simulink model "PCS"  (Simulink 8.0)
settings: Solver=ode23  StartTime=0.0  StopTime=0.3  RelTol=1e-3
undefined symbols (not defined in the file or in its folder): DiscIntNeverNeededParam, Ion, Lithium
libraries: powerlib x54, simulink x4, electricdrivelib x1, powerlib_extras x1
settings Model: Creator=wzhenh  LastModifiedBy=Administrator
settings SolverCC: ZeroCrossControl=DisableAll
settings DebuggingCC: FrameProcessingCompatibilityMsg=error
settings CodeAppCC: CustomSymbolStrType=$N$R$M_T  InternalIdentifier=Shortened
settings GRTTargetCC: CodeReplacementLibrary=None  CPPClassGenCompliant=on

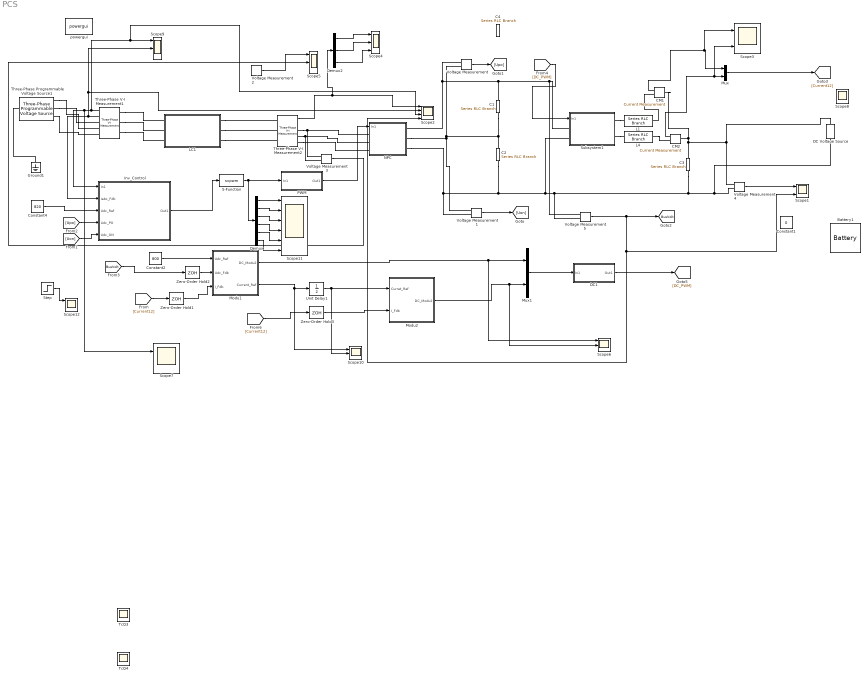
== system PCS ==
  Battery1 : electricdrivelib/Extra Sources/Battery  BatType=Lithium-Ion  ShowDetailedParameters=off  NomV=450  NomQ=2.5  SOC=20  PresetModel=off  MaxQ=2.625  FullV=2357.0739  Dis_rate=0.027175  R=1.8  Normal_OP=0.0565225  expZone=[2187.7812 0.0030706525]  Dis_Char=off  current=[1.5 3]  Units=Ampere-hour  Batt_Tr=30
  C1 : powerlib/Elements/Series RLC Branch  LConnTagsString=__new0  RConnTagsString=__new0  BranchType=C  Resistance=0.05  Inductance=22e-3  SetiL0=off  InitialCurrent=0  Capacitance=4110e-6  Setx0=on  InitialVoltage=480/1.732*1.414/2  Measurements=None
  C2 : powerlib/Elements/Series RLC Branch  LConnTagsString=__new0  RConnTagsString=__new0  BranchType=C  Resistance=0.05  Inductance=22e-3  SetiL0=off  InitialCurrent=0  Capacitance=4110e-6  Setx0=on  InitialVoltage=480/1.732*1.414/2  Measurements=None
  C3 : powerlib/Elements/Series RLC Branch  LConnTagsString=__new0  RConnTagsString=__new0  BranchType=RC  Resistance=0.05  Inductance=22e-3  SetiL0=off  InitialCurrent=0  Capacitance=120e-6  Setx0=off  InitialVoltage=400  Measurements=None
  C4 : powerlib/Elements/Series RLC Branch  LConnTagsString=__new0  RConnTagsString=__new0  BranchType=C  Resistance=0.05  Inductance=22e-3  SetiL0=off  InitialCurrent=0  Capacitance=4110e-6  Setx0=off  InitialVoltage=400  Measurements=None
  CM1 : powerlib/Measurements/Current Measurement  PhasorSimulation=off  OutputType=Complex  PSBequivalent=0
  CM2 : powerlib/Measurements/Current Measurement  PhasorSimulation=off  OutputType=Complex  PSBequivalent=0
  Constant1 : Constant  Value=0
  Constant2 : Constant  Value=800
  Constant4 : Constant  Value=820
  DC Voltage Source : powerlib/Electrical Sources/DC Voltage Source  Amplitude=450  Measurements=None
  DC1 : Subsystem
      mask init:
      | Dc_Pwm=7.8125e-6/5
  Demux : Demux  Outputs=6
  Demux2 : Demux  Outputs=3
  Ground1 : powerlib/Elements/Ground  LConnTagsString=a
  Inv_Control : Subsystem
  L1 : powerlib/Elements/Series RLC Branch  LConnTagsString=__new0  RConnTagsString=__new0  BranchType=L  Resistance=1  Inductance=1e-3  SetiL0=off  InitialCurrent=20  Capacitance=1e-6  Setx0=off  InitialVoltage=0  Measurements=None
  L4 : powerlib/Elements/Series RLC Branch  LConnTagsString=__new0  RConnTagsString=__new0  BranchType=L  Resistance=1  Inductance=1e-3  SetiL0=off  InitialCurrent=20  Capacitance=1e-6  Setx0=off  InitialVoltage=0  Measurements=None
  LC1 : Subsystem
  Modu1 : Subsystem
      mask init:
      | Ts_Dc=62.5e-6
  Modu2 : Subsystem
      mask init:
      | Ts_Dc=62.5e-6
  Mux : Mux  Inputs=2
  Mux1 : Mux  Inputs=2
  NPC : Subsystem
  PWM : Subsystem
      mask init:
      | Ts_Pwm=1.5625e-6
  S-Function : S-Function  FunctionName=svpwm  EnableBusSupport=off
  Scope{1,4..6,8..10,12} (8 alike) : Scope  NumInputPorts=3
      Scope4 settings: YMin=-5~-5~-5  YMax=5~5~5
  Scope11 : Scope  NumInputPorts=6
  Scope2 : Scope  NumInputPorts=4
      settings: YMin=-1000~-15~-400~799  YMax=1000~15~400~803.5
  Scope3 : Scope  NumInputPorts=2
      settings: YMin=-5~-5  YMax=5~5
  Scope7 : Scope  NumInputPorts=2
  Step : Step  Time=0.2  Before=780  After=820  SampleTime=62.5e-6
  Subsystem1 : Subsystem
  TcQ3 : Scope
  TcQ4 : Scope
  Three-Phase Programmable Voltage Source1 : powerlib/Electrical Sources/Three-Phase Programmable Voltage Source  PositiveSequence=[480 0 50]  VariationEntity=None  VariationType=Table of time-amplitude pairs  VariationTypeAlt=Step  VariationStep=0.5  VariationRate=10  VariationMagnitude=0.3  VariationFrequency=2  VariationTiming=[1 2]  VariationPhaseA=off  Amplitudes=[1 0.8 1.2 1.0]  TimeValues=[0 0.1 0.15 0.2]  HarmonicGeneration=off  HarmonicA=[3 0.2 -25 0]  HarmonicB=[2 0.15 35 2]  Timing="[0.05  3]"  BusType=swing  Pref=0  Qref=0  Qmin=-inf  Qmax=inf
  Three-Phase V-I Measurement1 : powerlib/Measurements/Three-Phase V-I Measurement  VoltageMeasurement=phase-to-ground  SetLabelV=off  LabelV=Vabc  Vpu=off  VpuLL=off  CurrentMeasurement=yes  SetLabelI=off  LabelI=Iabc  Ipu=off  Pbase=30000  Vbase=480  OutputType=Complex  PhasorSimulation=off  PSBequivalent=0
  Three-Phase V-I Measurement2 : powerlib/Measurements/Three-Phase V-I Measurement  VoltageMeasurement=phase-to-phase  SetLabelV=off  LabelV=Vabc  Vpu=off  VpuLL=off  CurrentMeasurement=yes  SetLabelI=off  LabelI=Iabc  Ipu=off  Pbase=30000  Vbase=480  OutputType=Complex  PhasorSimulation=off  PSBequivalent=0
  Unit Delay1 : UnitDelay  SampleTime=31.125e-6
  Voltage Measurement{,1..5} (6 alike) : powerlib/Measurements/Voltage Measurement  PhasorSimulation=off  OutputType=Complex  PSBequivalent=0
  Zero-Order Hold1 : ZeroOrderHold  SampleTime=62.5e-6
  Zero-Order Hold2 : ZeroOrderHold  SampleTime=125e-6
  Zero-Order Hold3 : ZeroOrderHold  SampleTime=62.5e-6
  powergui : powerlib/powergui  Priority=1  SimulationMode=Discrete  SolverType=Tustin  SampleTime=62.5e-6/32  frequency=60  SPID=off  DisableSnubberDevices=off  DisableRonSwitches=off  DisableVfSwitches=off  SwTol=0  Interpol=off  DisplayEquations=off  FunctionMessages=off  frequencyindice=0  Pbase=30000e3  ErrMax=1e-4  Iterations=50  UnitsV=kV  UnitsW=MW  echomessages=off  HookPort=off  EnableUseOfTLC=off  x0status=blocks  RestoreLinks=warning  ResistiveCurrentMeasurement=off  Frange=[0:2:500]  Ylog=off  Xlog=on  ShowGrid=off  save=off  variable=ZData  structure=psbbridges_str  ZoomFFT=off  StartTime=0.0  cycles=1  DisplayStyle=1  fundamental=50  FreqAxis=off  MaxFrequency=1000  frequencyindicesteady=1  RmsSteady=1  display=off  Ts=0  methode=off
  tag scope: BusVolt=global
  wires:
  Voltage Measurement/1 -> [Upo]
  Voltage Measurement1/1 -> [Uon]
  ? -> TcQ4/1
  ? -> TcQ3/1
  PWM/1(Out1) -> NPC/1(In1)
  [Uon] -> Inv_Control/5(Udc_ON)
  [Upo] -> Inv_Control/4(Udc_PO)
  Three-Phase V-I Measurement2/1 -> Demux2/1, Scope2/1
  S-Function/1 -> Demux/1, PWM/1(In1)
  Demux2/1 -> Scope4/1
  Demux2/2 -> Scope4/2
  Demux2/3 -> Scope4/3
  Voltage Measurement2/1 -> Scope5/1
  Voltage Measurement3/1 -> Scope5/2
  Inv_Control/1(Out1) -> S-Function/1
  Three-Phase V-I Measurement1/1 -> Scope2/3, Scope9/1, Scope7/1, Inv_Control/1(In1)
  Three-Phase V-I Measurement1/2 -> Scope2/2, Scope9/2, Inv_Control/2(Iabc_Fdb)
  [Current12] -> Zero-Order Hold1/1
  [Current12] -> Zero-Order Hold3/1
  Constant2/1 -> Modu1/1(Udc_Ref)
  Zero-Order Hold2/1 -> Modu1/2(Udc_Fdb)
  Zero-Order Hold1/1 -> Modu1/3(I_Fdb)
  Zero-Order Hold3/1 -> Modu2/2(I_Fdb)
  Modu1/2(Current_Ref) -> Scope10/1, Unit Delay1/1
  Unit Delay1/1 -> Modu2/1(Curret_Ref), Scope10/2
  [DC_PWM] -> Subsystem1/1(In1)
  Voltage Measurement4/1 -> Scope1/1
  Modu1/1(DC_Modu2) -> Scope6/1, Mux1/1
  Modu2/1(DC_Modu2) -> Scope6/2, Mux1/2
  Mux1/1 -> DC1/1(In1)
  DC1/1(Out1) -> [DC_PWM]
  [BusVolt] -> Zero-Order Hold2/1
  Voltage Measurement5/1 -> Scope2/4, Scope1/3, [BusVolt]
  CM1/1 -> Scope3/1, Mux/1
  CM2/1 -> Scope3/2, Mux/2
  Mux/1 -> [Current12]
  Demux/1 -> Scope11/1
  Demux/2 -> Scope11/2
  Demux/3 -> Scope11/3
  Demux/4 -> Scope11/4
  Demux/5 -> Scope11/5
  Demux/6 -> Scope11/6
  Step/1 -> Scope12/1
  Constant4/1 -> Inv_Control/3(Udc_Ref)
  connections:
  Three-Phase V-I Measurement2/RConn1 -- Voltage Measurement3/LConn1 -- NPC/LConn1
  Three-Phase V-I Measurement2/RConn2 -- Voltage Measurement3/LConn2 -- NPC/LConn2
  Ground1/LConn1 -- Three-Phase Programmable Voltage Source1/LConn1
  Three-Phase V-I Measurement2/RConn3 -- NPC/LConn3
  LC1/RConn1 -- Three-Phase V-I Measurement2/LConn1
  LC1/RConn2 -- Three-Phase V-I Measurement2/LConn2
  LC1/RConn3 -- Three-Phase V-I Measurement2/LConn3
  Three-Phase Programmable Voltage Source1/RConn1 -- Three-Phase V-I Measurement1/RConn1
  Three-Phase Programmable Voltage Source1/RConn2 -- Three-Phase V-I Measurement1/RConn2
  Three-Phase Programmable Voltage Source1/RConn3 -- Three-Phase V-I Measurement1/RConn3
  Three-Phase V-I Measurement1/LConn1 -- LC1/LConn1
  Three-Phase V-I Measurement1/LConn2 -- LC1/LConn2
  Three-Phase V-I Measurement1/LConn3 -- LC1/LConn3
  Subsystem1/RConn2 -- L4/LConn1
  Subsystem1/RConn1 -- L1/LConn1
  C3/LConn1 -- CM1/LConn1 -- CM2/LConn1 -- DC Voltage Source/RConn1 -- Voltage Measurement4/LConn1
  L1/RConn1 -- CM1/RConn1
  C1/LConn1 -- Voltage Measurement5/LConn1 -- Subsystem1/LConn1 -- NPC/RConn1 -- Voltage Measurement/LConn1
  Voltage Measurement/LConn2 -- Voltage Measurement1/LConn1 -- NPC/RConn2 -- C2/LConn1 -- C1/RConn1
  C3/RConn1 -- Subsystem1/LConn2 -- C2/RConn1 -- Voltage Measurement1/LConn2 -- NPC/RConn3 -- Voltage Measurement5/LConn2 -- DC Voltage Source/LConn1 -- Voltage Measurement4/LConn2
  L4/RConn1 -- CM2/RConn1

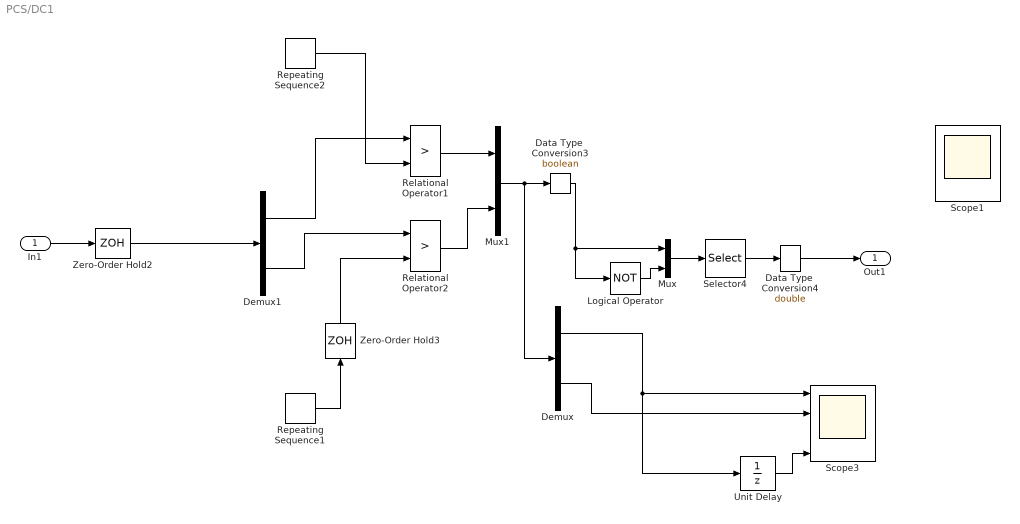
== system PCS/DC1 ==
  In1 : Inport
  Data Type  Conversion3 : DataTypeConversion  OutDataTypeStr=boolean  SampleTime=Dc_Pwm  SaturateOnIntegerOverflow=on  RndMeth=Zero
  Data Type  Conversion4 : DataTypeConversion  OutDataTypeStr=double  SampleTime=Dc_Pwm  SaturateOnIntegerOverflow=on  RndMeth=Zero
  Demux : Demux  Outputs=2
  Demux1 : Demux  Outputs=2
  Logical Operator : Logic  Operator=NOT  AllPortsSameDT=off  OutDataTypeStr=boolean  SampleTime=Dc_Pwm
  Mux : Mux  Inputs=2
  Mux1 : Mux  Inputs=2
  Relational Operator1 : RelationalOperator  Operator=>  SampleTime=Dc_Pwm  InputSameDT=on
  Relational Operator2 : RelationalOperator  Operator=>  SampleTime=Dc_Pwm  InputSameDT=on
  Repeating Sequence1 : simulink/Sources/Repeating Sequence  rep_seq_t=[0 62.5e-6 125e-6]  rep_seq_y=[1 0 1]
  Repeating Sequence2 : simulink/Sources/Repeating Sequence  rep_seq_t=[0 62.5e-6 125e-6]  rep_seq_y=[0 1 0]
  Scope1 : Scope  NumInputPorts=4
  Scope3 : Scope  NumInputPorts=4
  Selector4 : Selector  InputPortWidth=4  IndexOptions=Index vector (dialog)  Indices=[1 3 2 4]  OutputSizes=1
  Unit Delay : UnitDelay  SampleTime=Dc_Pwm
  Zero-Order Hold2 : ZeroOrderHold  SampleTime=Dc_Pwm
  Zero-Order Hold3 : ZeroOrderHold  SampleTime=Dc_Pwm
  Out1 : Outport
  wires:
  In1/1 -> Zero-Order Hold2/1
  Repeating Sequence1/1 -> Zero-Order Hold3/1
  Zero-Order Hold3/1 -> Relational Operator2/2
  Data Type  Conversion4/1 -> Out1/1
  Demux/1 -> Unit Delay/1, Scope3/1
  Demux/2 -> Scope3/2
  Selector4/1 -> Data Type  Conversion4/1
  Data Type  Conversion3/1 -> Mux/1, Logical Operator/1
  Logical Operator/1 -> Mux/2
  Mux/1 -> Selector4/1
  Unit Delay/1 -> Scope3/4
  Repeating Sequence2/1 -> Relational Operator1/2
  Zero-Order Hold2/1 -> Demux1/1
  Demux1/1 -> Relational Operator1/1
  Demux1/2 -> Relational Operator2/1
  Mux1/1 -> Demux/1, Data Type  Conversion3/1
  Relational Operator1/1 -> Mux1/1
  Relational Operator2/1 -> Mux1/2

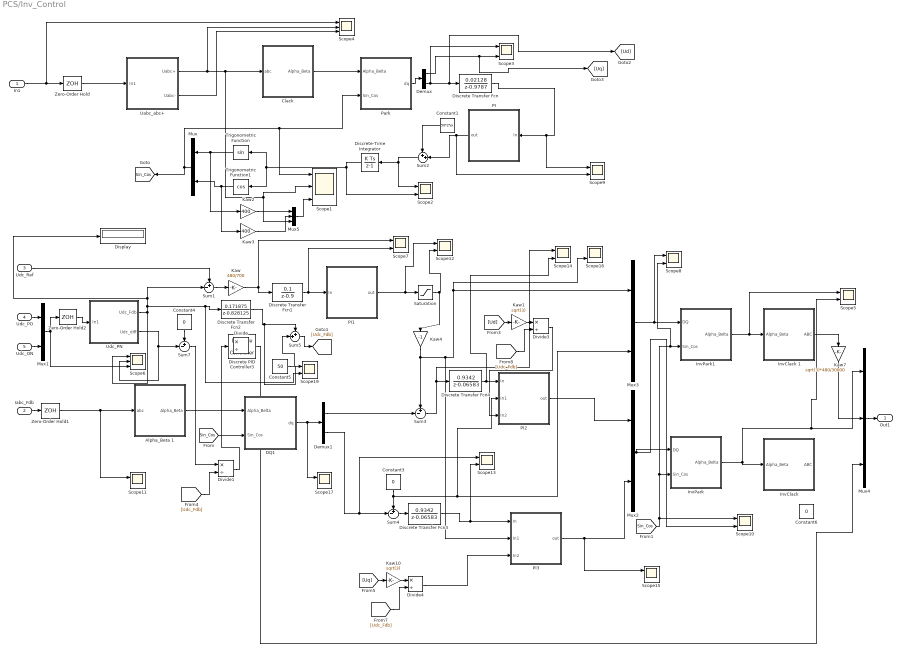
== system PCS/Inv_Control ==
  In1 : Inport
  Iabc_Fdb : Inport  Port=2
  Udc_Ref : Inport  Port=3
  Udc_PO : Inport  Port=4
  Udc_ON : Inport  Port=5
  Alpha_Beta 1 : Subsystem
      mask init:
      | Ts_PLL=125e-6
  "Clack " : Subsystem
      mask init:
      | Ts_PLL=125e-6
  Constant1 : Constant  Value=50*2*pi
  Constant3 : Constant  Value=0
  Constant4 : Constant  Value=0
  Constant5 : Constant  Value=50
  Constant6 : Constant  Value=0
  DQ1 : Subsystem
      mask init:
      | Ts_PLL=125e-6
  Demux : Demux  Outputs=2
  Demux1 : Demux  Outputs=2
  Discrete PID Controller3 : powerlib_extras/Discrete  Control Blocks/Discrete PID Controller  Kp=3.0234375  Ki=31.25  Kd=0  TcD=0  Par_Limits=[16384 -16384]  Init=0  Ts=125e-6
  Discrete Transfer Fcn : DiscreteTransferFcn  Numerator=[0.02128]  Denominator=[1 -0.9787]  SampleTime=125e-6
  Discrete Transfer Fcn1 : DiscreteTransferFcn  Numerator=[0.1]  Denominator=[1 -0.9]  SampleTime=125e-6
  Discrete Transfer Fcn2 : DiscreteTransferFcn  Numerator=[0.171875]  Denominator=[1 -0.828125]  SampleTime=20e-6
  Discrete Transfer Fcn3 : DiscreteTransferFcn  Numerator=[0.9342]  Denominator=[1 -0.06583]  SampleTime=125e-6
  Discrete Transfer Fcn4 : DiscreteTransferFcn  Numerator=[0.9342]  Denominator=[1 -0.06583]  SampleTime=125e-6
  Discrete-Time Integrator : DiscreteIntegrator  gainval=1  SampleTime=125e-6  UpperSaturationLimit=1.2  LowerSaturationLimit=-1.2  ICPrevOutput=DiscIntNeverNeededParam  ICPrevScaledInput=DiscIntNeverNeededParam
  Display : Display
  Divide{,1,3..4} (4 alike) : Product  Inputs=*/
  "InvClack " : Subsystem
      mask init:
      | Ts_PLL=125e-6
  InvClack 1 : Subsystem
      mask init:
      | Ts_PLL=125e-6
  InvPark : Subsystem
      mask init:
      | Ts_PLL=125e-6
  InvPark1 : Subsystem
      mask init:
      | Ts_PLL=125e-6
  Kaw : Gain  DisableCoverage=on  Gain=480/700  SampleTime=125e-6
  Kaw1 : Gain  DisableCoverage=on  Gain=sqrt(3)  SampleTime=125e-6
  Kaw10 : Gain  DisableCoverage=on  Gain=sqrt(3)  SampleTime=125e-6
  Kaw2 : Gain  DisableCoverage=on  Gain=400  SampleTime=125e-6
  Kaw3 : Gain  DisableCoverage=on  Gain=400  SampleTime=125e-6
  Kaw4 : Gain  DisableCoverage=on  Gain=-1  SampleTime=125e-6
  Kaw7 : Gain  DisableCoverage=on  Gain=sqrt(3)*480/30000  SampleTime=125e-6
  Mux{,1..3} (4 alike) : Mux  Inputs=2
  Mux4 : Mux  Inputs=3
  Mux5 : Mux  Inputs=3
      settings: DisplayOption=signals
  PI : Subsystem  SystemSampleTime=Ts  mask{Kp=0.32257080078125, Ki=14.6484375, Kaw=45.8984375, Ts=125e-6}
      mask prompts: Ts "Sample time (-1 for inherited):"
      mask init:
      | Ts=125e-6
      mask TypeOptions Kp: Kp/Gain
      mask TypeOptions Ki: Ki/Gain
      mask TypeOptions Kaw: Kaw/Gain
      mask TypeOptions Ts: Integral Gain/SampleTime | Integral Gain1/SampleTime | Integrator/SampleTime | Proportional Gain/SampleTime | Sum/SampleTime | Sum1/SampleTime | Sum2/SampleTime | SystemSampleTime
  PI1 : Subsystem  SystemSampleTime=Ts  mask{Kp=1.256591796875, Ki=23.54038011, Kaw=18.73283928, Ts=125e-6, UpperLimit=4.8, LowerLimit=-4.8}
      mask prompts: Ts "Sample time (-1 for inherited):"; UpperLimit "Upper limit:"; LowerLimit "Lower limit:"
      mask init:
      | Ts=125e-6
      mask TypeOptions Kp: Kp/Gain
      mask TypeOptions Ki: Ki/Gain
      mask TypeOptions Kaw: Kaw/Gain
      mask TypeOptions Ts: Integral Gain/SampleTime | Integral Gain1/SampleTime | Integrator/SampleTime | Proportional Gain/SampleTime | Sum/SampleTime | Sum1/SampleTime | Sum2/SampleTime | SystemSampleTime
      mask TypeOptions UpperLimit: Saturation/UpperLimit
      mask TypeOptions LowerLimit: Saturation/LowerLimit
  PI2 : Subsystem  SystemSampleTime=Ts  mask{Kp=2.3876953125, Ki=692.9034009, Kaw=290.2078983, Ts=125e-6, UpperLimit=1, LowerLimit=-1}
      mask prompts: Ts "Sample time (-1 for inherited):"; UpperLimit "Upper limit:"; LowerLimit "Lower limit:"
      mask init:
      | Ts=125e-6
      mask TypeOptions Kp: Kp/Gain
      mask TypeOptions Ki: Ki/Gain
      mask TypeOptions Kaw: Kaw/Gain
      mask TypeOptions Ts: Integral Gain/SampleTime | Integral Gain1/SampleTime | Integrator/SampleTime | Proportional Gain/SampleTime | Sum/SampleTime | Sum1/SampleTime | Sum2/SampleTime | SystemSampleTime
      mask TypeOptions UpperLimit: Saturation/UpperLimit
      mask TypeOptions LowerLimit: Saturation/LowerLimit
  PI3 : Subsystem  SystemSampleTime=Ts  mask{Kp=2.3876953125, Ki=692.9034009, Kaw=290.2078983, Ts=125e-6, UpperLimit=1, LowerLimit=-1}
      mask prompts: Ts "Sample time (-1 for inherited):"; UpperLimit "Upper limit:"; LowerLimit "Lower limit:"
      mask init:
      | Ts=125e-6
      mask TypeOptions Kp: Kp/Gain
      mask TypeOptions Ki: Ki/Gain
      mask TypeOptions Kaw: Kaw/Gain
      mask TypeOptions Ts: Integral Gain/SampleTime | Integral Gain1/SampleTime | Integrator/SampleTime | Proportional Gain/SampleTime | Sum/SampleTime | Sum1/SampleTime | Sum2/SampleTime | SystemSampleTime
      mask TypeOptions UpperLimit: Saturation/UpperLimit
      mask TypeOptions LowerLimit: Saturation/LowerLimit
  Park : Subsystem
      mask init:
      | Ts_PLL=125e-6
  Saturation : Saturate  UpperLimit=51  LowerLimit=-51  SampleTime=125e-6
  Scope{1,3..4,6} (4 alike) : Scope  NumInputPorts=3
  Scope{2,5,7..17,19} (14 alike) : Scope  NumInputPorts=2
  Sum{1,3..4,7} (4 alike) : Sum  Inputs=+-|  SampleTime=125e-6
  Sum2 : Sum  Inputs=++|  SampleTime=125e-6
  Sum5 : Sum  Inputs=++|  SampleTime=125e-6
  Trigonometric Function : Trigonometry  SampleTime=125e-6
  Trigonometric Function1 : Trigonometry  Operator=cos  SampleTime=125e-6
  Uabc_abc+ : Subsystem
      mask init:
      | Ts_PLL=125e-6
  Udc_PN : Subsystem
      mask init:
      | Ts_PLL=125e-6
  Zero-Order Hold : ZeroOrderHold  SampleTime=125e-6
  Zero-Order Hold1 : ZeroOrderHold  SampleTime=125e-6
  Zero-Order Hold2 : ZeroOrderHold  SampleTime=125e-6
  Out1 : Outport
  tag scope: Sin_Cos=global
  wires:
  In1/1 -> Scope4/1, Zero-Order Hold/1
  Zero-Order Hold/1 -> Uabc_abc+/1(In1)
  Uabc_abc+/1(Uabc+) -> Scope4/2, Mux5/3, Scope1/2, "Clack "/1(abc)
  "Clack "/1(Alpha_Beta) -> Park/1(Alpha_Belta)
  Trigonometric Function/1 -> Kaw2/1, Mux/1
  Trigonometric Function1/1 -> Kaw3/1, Mux/2
  Mux/1 -> Park/2(Sin_Cos), Scope1/1, [Sin_Cos]
  Park/1(dq) -> Demux/1
  Demux/1 -> [Uq], Scope3/3
  Demux/2 -> [Ud], Discrete Transfer Fcn/1, Scope3/1
  Discrete-Time Integrator/1 -> Trigonometric Function/1, Trigonometric Function1/1, Scope2/2
  Sum2/1 -> Scope2/1, Discrete-Time Integrator/1
  PI/1(out) -> Scope9/2, Sum2/2
  Alpha_Beta 1/1(Alpha_Beta) -> DQ1/1(Alpha_Belta)
  [Sin_Cos] -> DQ1/2(Sin_Cos)
  Udc_PO/1 -> Mux1/1
  Udc_ON/1 -> Mux1/2
  Mux1/1 -> Zero-Order Hold2/1, Scope6/3
  Udc_Ref/1 -> Sum1/1
  Udc_PN/1(Udc_Fdb) -> Scope6/1, Sum1/2, Display/1, Scope19/2, Discrete Transfer Fcn2/1
  Discrete Transfer Fcn1/1 -> PI1/1(In), Scope7/2
  PI1/1(out) -> Scope12/1, Saturation/1
  DQ1/1(dq) -> Scope17/1, Demux1/1
  Sum4/1 -> Discrete Transfer Fcn3/1
  Discrete Transfer Fcn3/1 -> Scope13/2, PI3/1(In)
  Mux2/1 -> Scope10/2, InvPark/1(DQ)
  [Sin_Cos] -> InvPark/2(Sin_Cos), Scope8/2, InvPark1/2(Sin_Cos), Scope10/1
  InvPark/1(Alpha_Belta) -> "InvClack "/1(Alpha_Beta), Scope5/2, Mux4/1
  Mux3/1 -> Scope8/1, InvPark1/1(DQ)
  InvPark1/1(Alpha_Belta) -> Scope5/1, InvClack 1/1(Alpha_Beta)
  InvClack 1/1(ABC) -> Kaw7/1
  Udc_PN/2(Udc_diff) -> Scope6/2, Sum7/2
  Constant4/1 -> Sum7/1
  Mux4/1 -> Out1/1
  Constant3/1 -> PI2/2(In1), Mux3/2, Sum4/1
  Iabc_Fdb/1 -> Zero-Order Hold1/1
  Zero-Order Hold1/1 -> Scope11/1, Alpha_Beta 1/1(abc)
  Discrete Transfer Fcn/1 -> Scope9/1, PI/1(In)
  Sum3/1 -> Scope14/1, Discrete Transfer Fcn4/1
  Demux1/1 -> Sum3/2
  Demux1/2 -> Sum4/2, Scope13/1
  Kaw7/1 -> Mux4/2
  Kaw4/1 -> PI3/2(In1), Scope16/2, Mux3/1, Sum3/1
  Sum1/1 -> Kaw/1
  Kaw/1 -> Discrete Transfer Fcn1/1, Scope7/1
  Kaw10/1 -> Divide4/1
  [Udc_Fdb] -> Divide4/2
  [Uq] -> Kaw10/1
  Zero-Order Hold2/1 -> Udc_PN/1(In1)
  PI3/1(out) -> Scope15/1, Mux2/2
  Discrete Transfer Fcn4/1 -> Scope14/2, PI2/1(In)
  Kaw1/1 -> Divide3/1
  [Udc_Fdb] -> Divide3/2
  [Ud] -> Kaw1/1
  PI2/1(out) -> Mux2/1
  Saturation/1 -> Kaw4/1, Scope12/2
  Divide4/1 -> PI3/3(In2)
  Divide3/1 -> PI2/3(In2)
  Discrete Transfer Fcn2/1 -> Sum5/1, Scope19/1
  Constant5/1 -> Sum5/2
  Sum5/1 -> [Udc_Fdb]
  Discrete PID Controller3/1 -> Mux4/3
  Sum7/1 -> Divide1/1
  [Udc_Fdb] -> Divide1/2
  Divide1/1 -> Discrete PID Controller3/1
  Constant1/1 -> Sum2/1
  Uabc_abc+/2(Uabc-) -> Scope4/3
  Mux5/1 -> Scope1/3
  Kaw2/1 -> Mux5/1
  Kaw3/1 -> Mux5/2

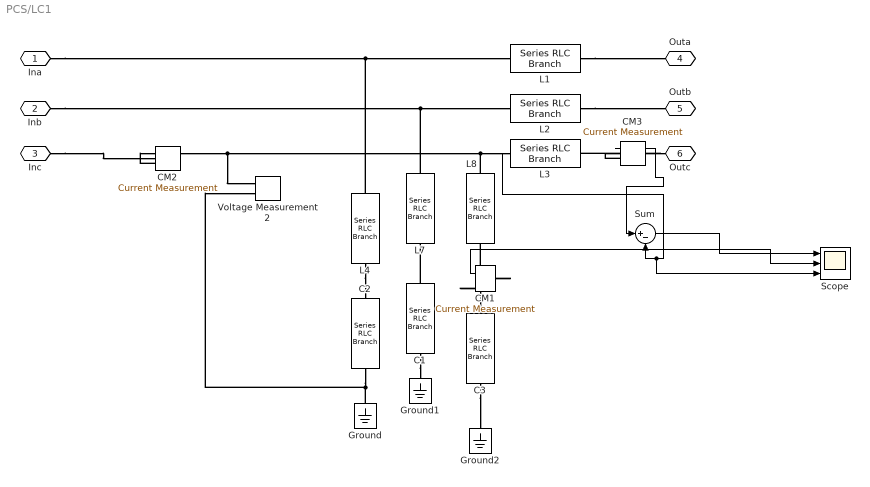
== system PCS/LC1 ==
  C1 : powerlib/Elements/Series RLC Branch  LConnTagsString=__new0  RConnTagsString=__new0  BranchType=C  Resistance=1  Inductance=22e-3  SetiL0=off  InitialCurrent=0  Capacitance=22e-6  Setx0=off  InitialVoltage=480/1.732*1.414  Measurements=None
  C2 : powerlib/Elements/Series RLC Branch  LConnTagsString=__new0  RConnTagsString=__new0  BranchType=C  Resistance=1  Inductance=22e-3  SetiL0=off  InitialCurrent=0  Capacitance=22e-6  Setx0=off  InitialVoltage=480/1.732*1.414  Measurements=None
  C3 : powerlib/Elements/Series RLC Branch  LConnTagsString=__new0  RConnTagsString=__new0  BranchType=C  Resistance=1  Inductance=22e-3  SetiL0=off  InitialCurrent=0  Capacitance=22e-6  Setx0=off  InitialVoltage=480/1.732*1.414  Measurements=None
  CM1 : powerlib/Measurements/Current Measurement  PhasorSimulation=off  OutputType=Complex  PSBequivalent=0
  CM2 : powerlib/Measurements/Current Measurement  PhasorSimulation=off  OutputType=Complex  PSBequivalent=0
  CM3 : powerlib/Measurements/Current Measurement  PhasorSimulation=off  OutputType=Complex  PSBequivalent=0
  Ground : powerlib/Elements/Ground  LConnTagsString=a
  Ground1 : powerlib/Elements/Ground  LConnTagsString=a
  Ground2 : powerlib/Elements/Ground  LConnTagsString=a
  L1 : powerlib/Elements/Series RLC Branch  LConnTagsString=__new0  RConnTagsString=__new0  BranchType=L  Resistance=1  Inductance=760e-6  SetiL0=off  InitialCurrent=0  Capacitance=1e-6  Setx0=off  InitialVoltage=0  Measurements=None
  L2 : powerlib/Elements/Series RLC Branch  LConnTagsString=__new0  RConnTagsString=__new0  BranchType=L  Resistance=1  Inductance=760e-6  SetiL0=off  InitialCurrent=0  Capacitance=1e-6  Setx0=off  InitialVoltage=0  Measurements=None
  L3 : powerlib/Elements/Series RLC Branch  LConnTagsString=__new0  RConnTagsString=__new0  BranchType=L  Resistance=1  Inductance=760e-6  SetiL0=off  InitialCurrent=0  Capacitance=1e-6  Setx0=off  InitialVoltage=0  Measurements=None
  L4 : powerlib/Elements/Series RLC Branch  LConnTagsString=__new0  RConnTagsString=__new0  BranchType=R  Resistance=0.05  Inductance=22e-3  SetiL0=off  InitialCurrent=0  Capacitance=1e-6  Setx0=off  InitialVoltage=0  Measurements=None
  L7 : powerlib/Elements/Series RLC Branch  LConnTagsString=__new0  RConnTagsString=__new0  BranchType=R  Resistance=0.05  Inductance=22e-3  SetiL0=off  InitialCurrent=0  Capacitance=1e-6  Setx0=off  InitialVoltage=0  Measurements=None
  L8 : powerlib/Elements/Series RLC Branch  LConnTagsString=__new0  RConnTagsString=__new0  BranchType=R  Resistance=0.05  Inductance=22e-3  SetiL0=off  InitialCurrent=0  Capacitance=1e-6  Setx0=off  InitialVoltage=0  Measurements=None
  Scope : Scope  NumInputPorts=3
  Sum : Sum  Inputs=|+-
  Voltage Measurement2 : powerlib/Measurements/Voltage Measurement  PhasorSimulation=off  OutputType=Complex  PSBequivalent=0
  Ina : PMIOPort  Port=1  Side=Left
  Inb : PMIOPort  Port=2  Side=Left
  Inc : PMIOPort  Port=3  Side=Left
  Outa : PMIOPort  Port=4  Side=Right
  Outb : PMIOPort  Port=5  Side=Right
  Outc : PMIOPort  Port=6  Side=Right
  wires:
  CM3/1 -> Sum/1
  CM2/1 -> Scope/3, Sum/2
  Sum/1 -> Scope/1
  CM1/1 -> Scope/2
  connections:
  L8/RConn1 -- Voltage Measurement2/LConn1 -- CM2/RConn1 -- L3/LConn1
  L7/RConn1 -- Inb/RConn1 -- L2/LConn1
  C3/LConn1 -- Ground2/LConn1
  C1/LConn1 -- Ground1/LConn1
  L2/RConn1 -- Outb/RConn1
  L1/RConn1 -- Outa/RConn1
  Ina/RConn1 -- L4/RConn1 -- L1/LConn1
  L4/LConn1 -- C2/LConn1
  C1/RConn1 -- L7/LConn1
  Inc/RConn1 -- CM2/LConn1
  CM3/LConn1 -- L3/RConn1
  CM3/RConn1 -- Outc/RConn1
  CM1/RConn1 -- L8/LConn1
  CM1/LConn1 -- C3/RConn1
  C2/RConn1 -- Ground/LConn1 -- Voltage Measurement2/LConn2

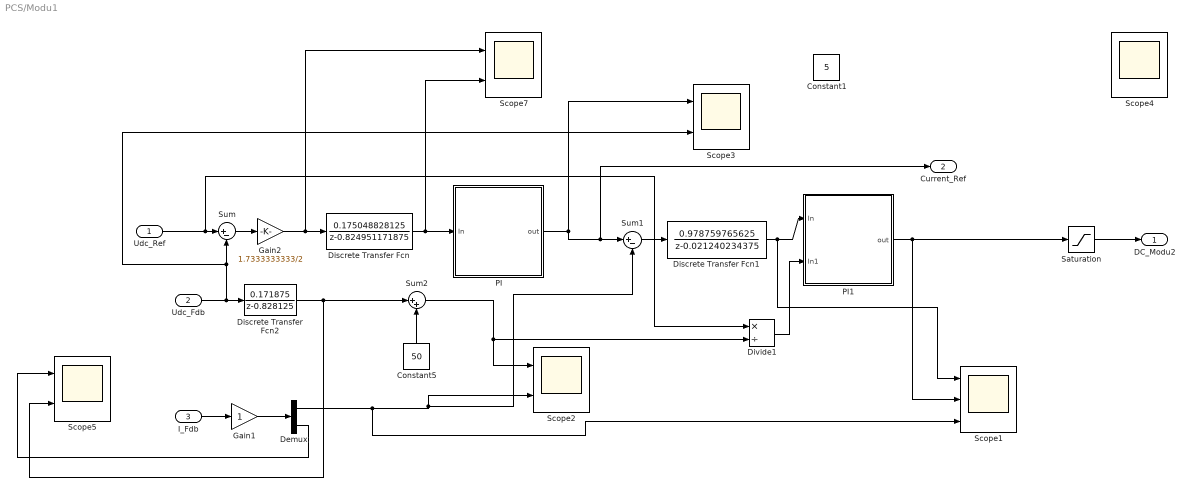
== system PCS/Modu1 ==
  Udc_Ref : Inport
  Udc_Fdb : Inport  Port=2
  I_Fdb : Inport  Port=3
  Constant1 : Constant  Value=5
  Constant5 : Constant  Value=50
  Demux : Demux  Outputs=2
  Discrete Transfer Fcn : DiscreteTransferFcn  Numerator=[0.175048828125]  Denominator=[1 -0.824951171875]  SampleTime=Ts_Dc
  Discrete Transfer Fcn1 : DiscreteTransferFcn  Numerator=[0.978759765625]  Denominator=[1 -0.021240234375]  SampleTime=Ts_Dc
  Discrete Transfer Fcn2 : DiscreteTransferFcn  Numerator=[0.171875]  Denominator=[1 -0.828125]  SampleTime=2000e-6
  Divide1 : Product  Inputs=*/
  Gain1 : Gain  SampleTime=Ts_Dc
  Gain2 : Gain  Gain=1.7333333333/2  SampleTime=Ts_Dc
  PI : Subsystem  SystemSampleTime=Ts  mask{Kp=1.256637061, Ki=12.8935972, Kaw=10.26039864, Ts=Ts_Dc, UpperLimit=70, LowerLimit=-70}
      mask prompts: Ts "Sample time (-1 for inherited):"; UpperLimit "Upper limit:"; LowerLimit "Lower limit:"
      mask init:
      | Ts=62.5e-6
      mask TypeOptions Kp: Kp/Gain
      mask TypeOptions Ki: Ki/Gain
      mask TypeOptions Kaw: Kaw/Gain
      mask TypeOptions Ts: Integral Gain/SampleTime | Integral Gain1/SampleTime | Integrator/SampleTime | Proportional Gain/SampleTime | Sum/SampleTime | Sum1/SampleTime | Sum2/SampleTime | SystemSampleTime
      mask TypeOptions UpperLimit: Saturation/UpperLimit
      mask TypeOptions LowerLimit: Saturation/LowerLimit
  PI1 : Subsystem  SystemSampleTime=Ts  mask{Kp=2.513274123*0.8, Ki=515.7438879, Kaw=205.2079728, Ts=Ts_Dc, UpperLimit=1, LowerLimit=-1}
      mask prompts: Ts "Sample time (-1 for inherited):"; UpperLimit "Upper limit:"; LowerLimit "Lower limit:"
      mask init:
      | Ts=62.5e-6
      mask TypeOptions Kp: Kp/Gain
      mask TypeOptions Ki: Ki/Gain
      mask TypeOptions Kaw: Kaw/Gain
      mask TypeOptions Ts: Integral Gain/SampleTime | Integral Gain1/SampleTime | Integrator/SampleTime | Proportional Gain/SampleTime | Sum/SampleTime | Sum1/SampleTime | Sum2/SampleTime | SystemSampleTime
      mask TypeOptions UpperLimit: Saturation/UpperLimit
      mask TypeOptions LowerLimit: Saturation/LowerLimit
  Saturation : Saturate  UpperLimit=0.9  LowerLimit=0.01  SampleTime=62.5e-6
  Scope1 : Scope  NumInputPorts=3
  Scope{2..5,7} (5 alike) : Scope  NumInputPorts=2
  Sum : Sum  Inputs=|+-  SampleTime=Ts_Dc
  Sum1 : Sum  Inputs=|+-  SampleTime=Ts_Dc
  Sum2 : Sum  Inputs=|++  SampleTime=Ts_Dc
  DC_Modu2 : Outport
  Current_Ref : Outport  Port=2
  wires:
  Udc_Ref/1 -> Divide1/1, Sum/1
  Discrete Transfer Fcn/1 -> Scope7/2, PI/1(In)
  I_Fdb/1 -> Gain1/1
  Sum1/1 -> Discrete Transfer Fcn1/1
  Discrete Transfer Fcn1/1 -> Scope1/1, PI1/1(In)
  Discrete Transfer Fcn2/1 -> Scope5/2, Sum2/1
  Sum2/1 -> Divide1/2, Scope2/1
  Constant5/1 -> Sum2/2
  Gain1/1 -> Demux/1
  Sum/1 -> Gain2/1
  Gain2/1 -> Scope7/1, Discrete Transfer Fcn/1
  PI1/1(out) -> Saturation/1, Scope1/2
  Udc_Fdb/1 -> Scope3/2, Sum/2, Discrete Transfer Fcn2/1
  Divide1/1 -> PI1/2(In1)
  Demux/1 -> Scope1/3, Sum1/2, Scope2/2
  Demux/2 -> Scope5/1
  Saturation/1 -> DC_Modu2/1
  PI/1(out) -> Scope3/1, Current_Ref/1, Sum1/1

== system PCS/Modu2 ==
  Curret_Ref : Inport
  I_Fdb : Inport  Port=2
  Constant1 : Constant  Value=0.5
  Demux : Demux  Outputs=2
  Discrete Transfer Fcn1 : DiscreteTransferFcn  Numerator=[0.978759765625]  Denominator=[1 -0.021240234375]  SampleTime=Ts_Dc
  PI1 : Subsystem  SystemSampleTime=Ts  mask{Kp=2.513274123, Ki=515.7438879, Kaw=205.2079728, Ts=Ts_Dc, UpperLimit=1, LowerLimit=-1}
      mask prompts: Ts "Sample time (-1 for inherited):"; UpperLimit "Upper limit:"; LowerLimit "Lower limit:"
      mask init:
      | Ts=125e-6
      mask TypeOptions Kp: Kp/Gain
      mask TypeOptions Ki: Ki/Gain
      mask TypeOptions Kaw: Kaw/Gain
      mask TypeOptions Ts: Integral Gain/SampleTime | Integral Gain1/SampleTime | Integrator/SampleTime | Proportional Gain/SampleTime | Sum/SampleTime | Sum1/SampleTime | Sum2/SampleTime | SystemSampleTime
      mask TypeOptions UpperLimit: Saturation/UpperLimit
      mask TypeOptions LowerLimit: Saturation/LowerLimit
  Saturation : Saturate  UpperLimit=0.9  LowerLimit=0.01  SampleTime=Ts_Dc
  Scope1 : Scope  NumInputPorts=3
  Scope2 : Scope  NumInputPorts=3
  Sum1 : Sum  Inputs=|+-  SampleTime=Ts_Dc
  DC_Modu2 : Outport
  wires:
  Discrete Transfer Fcn1/1 -> PI1/1(In)
  Sum1/1 -> Discrete Transfer Fcn1/1
  Curret_Ref/1 -> Scope1/1, Sum1/1
  I_Fdb/1 -> Demux/1
  PI1/1(out) -> Scope2/1, Saturation/1
  Demux/2 -> Scope1/2, Sum1/2
  Saturation/1 -> DC_Modu2/1

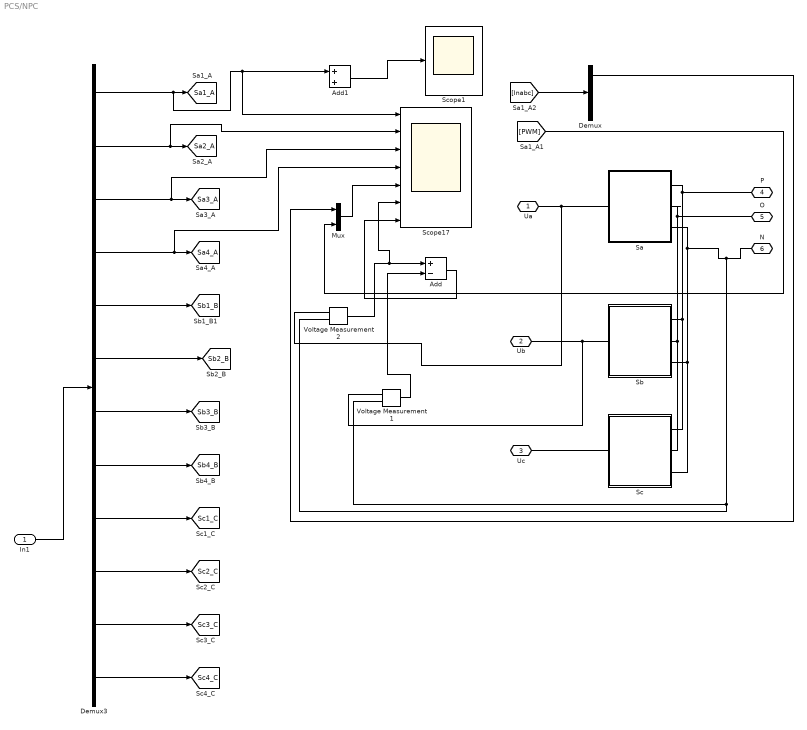
== system PCS/NPC ==
  In1 : Inport
  Add : Sum  Inputs=+-
  Add1 : Sum
  Demux : Demux  Outputs=3
  Demux3 : Demux  Outputs=12
  Mux : Mux  Inputs=2
  Sa : Subsystem
  Sb : Subsystem
  Sc : Subsystem
  Scope1 : Scope
  Scope17 : Scope  NumInputPorts=7
  Voltage Measurement1 : powerlib/Measurements/Voltage Measurement  PhasorSimulation=off  OutputType=Complex  PSBequivalent=0
  Voltage Measurement2 : powerlib/Measurements/Voltage Measurement  PhasorSimulation=off  OutputType=Complex  PSBequivalent=0
  Ua : PMIOPort  Port=1  Side=Left
  Ub : PMIOPort  Port=2  Side=Left
  Uc : PMIOPort  Port=3  Side=Left
  P : PMIOPort  Port=4  Side=Right
  O : PMIOPort  Port=5  Side=Right
  N : PMIOPort  Port=6  Side=Right
  tag scope: Sa1_A=global, Sa2_A=global, Sa3_A=global, Sa4_A=global, Sb1_B=global, Sb2_B=global, Sb3_B=global, Sb4_B=global, Sc1_C=global, Sc2_C=global, Sc3_C=global, Sc4_C=global
  wires:
  In1/1 -> Demux3/1
  Demux3/4 -> Scope17/4, [Sa4_A]
  Demux3/6 -> [Sb2_B]
  Demux3/7 -> [Sb3_B]
  Demux3/8 -> [Sb4_B]
  Demux3/9 -> [Sc1_C]
  Demux3/11 -> [Sc3_C]
  Demux3/12 -> [Sc4_C]
  Demux3/10 -> [Sc2_C]
  Voltage Measurement2/1 -> Scope17/6, Add/1
  Voltage Measurement1/1 -> Add/2
  Add/1 -> Scope17/7
  [PWM] -> Mux/2
  [Inabc] -> Demux/1
  Mux/1 -> Scope17/5
  Demux3/1 -> Scope17/1, Add1/1, [Sa1_A]
  Demux3/2 -> Scope17/2, [Sa2_A]
  Demux3/3 -> Scope17/3, [Sa3_A]
  Demux3/5 -> [Sb1_B]
  Add1/1 -> Scope1/1
  Demux/1 -> Mux/1
  connections:
  Sa/RConn2 -- O/RConn1 -- Sc/RConn2 -- Sb/RConn2
  Sb/RConn3 -- Sa/RConn3 -- Voltage Measurement2/LConn2 -- Voltage Measurement1/LConn2 -- N/RConn1 -- Sc/RConn3
  Sc/RConn1 -- Sa/RConn1 -- P/RConn1 -- Sb/RConn1
  Uc/RConn1 -- Sc/LConn1
  Ub/RConn1 -- Voltage Measurement1/LConn1 -- Sb/LConn1
  Ua/RConn1 -- Voltage Measurement2/LConn1 -- Sa/LConn1

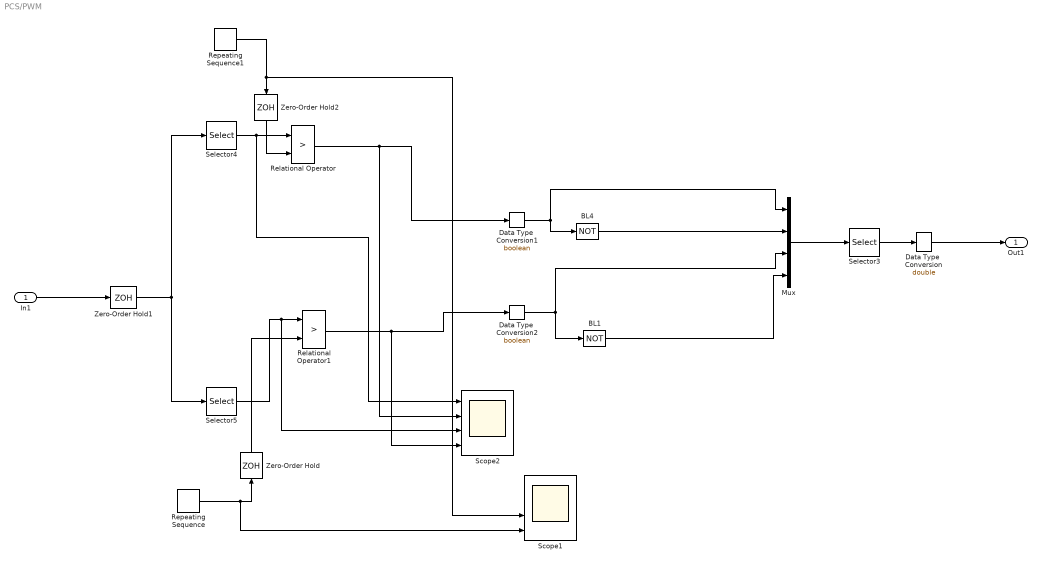
== system PCS/PWM ==
  In1 : Inport
  BL1 : Logic  Operator=NOT  Inputs=1  SampleTime=Ts_Pwm
  BL4 : Logic  Operator=NOT  Inputs=1  SampleTime=Ts_Pwm
  Data Type  Conversion : DataTypeConversion  OutDataTypeStr=double  SampleTime=Ts_Pwm  SaturateOnIntegerOverflow=on  RndMeth=Zero
  Data Type  Conversion1 : DataTypeConversion  OutDataTypeStr=boolean  SampleTime=Ts_Pwm  SaturateOnIntegerOverflow=on  RndMeth=Zero
  Data Type  Conversion2 : DataTypeConversion  OutDataTypeStr=boolean  SampleTime=Ts_Pwm  SaturateOnIntegerOverflow=on  RndMeth=Zero
  Mux : Mux
  Relational Operator : RelationalOperator  Operator=>  SampleTime=Ts_Pwm  InputSameDT=on
  Relational Operator1 : RelationalOperator  Operator=>  SampleTime=Ts_Pwm  InputSameDT=on
  Repeating Sequence : simulink/Sources/Repeating Sequence  rep_seq_t=[0 62.5e-6 125e-6]  rep_seq_y=[0 1 0]
  Repeating Sequence1 : simulink/Sources/Repeating Sequence  rep_seq_t=[0 62.5e-6 125e-6]  rep_seq_y=[1 0 1]
  Scope1 : Scope  NumInputPorts=4
  Scope2 : Scope  NumInputPorts=4
  Selector3 : Selector  InputPortWidth=12  IndexOptions=Index vector (dialog)  Indices=[1 10 4 7 2 11 5 8 3 12 6 9]  OutputSizes=1
  Selector4 : Selector  InputPortWidth=6  IndexOptions=Index vector (dialog)  Indices=[1 3 5]  OutputSizes=1
  Selector5 : Selector  InputPortWidth=6  IndexOptions=Index vector (dialog)  Indices=[2 4 6]  OutputSizes=1
  Zero-Order Hold : ZeroOrderHold  SampleTime=Ts_Pwm
  Zero-Order Hold1 : ZeroOrderHold  SampleTime=Ts_Pwm
  Zero-Order Hold2 : ZeroOrderHold  SampleTime=Ts_Pwm
  Out1 : Outport
  wires:
  In1/1 -> Zero-Order Hold1/1
  Selector3/1 -> Data Type  Conversion/1
  Data Type  Conversion/1 -> Out1/1
  BL4/1 -> Mux/2
  BL1/1 -> Mux/4
  Data Type  Conversion2/1 -> BL1/1, Mux/3
  Mux/1 -> Selector3/1
  Repeating Sequence/1 -> Zero-Order Hold/1, Scope1/4
  Zero-Order Hold1/1 -> Selector4/1, Selector5/1
  Selector4/1 -> Scope2/1, Relational Operator/1
  Selector5/1 -> Scope2/3, Relational Operator1/1
  Repeating Sequence1/1 -> Scope1/3, Zero-Order Hold2/1
  Zero-Order Hold/1 -> Relational Operator1/2
  Relational Operator1/1 -> Scope2/4, Data Type  Conversion2/1
  Relational Operator/1 -> Scope2/2, Data Type  Conversion1/1
  Data Type  Conversion1/1 -> BL4/1, Mux/1
  Zero-Order Hold2/1 -> Relational Operator/2

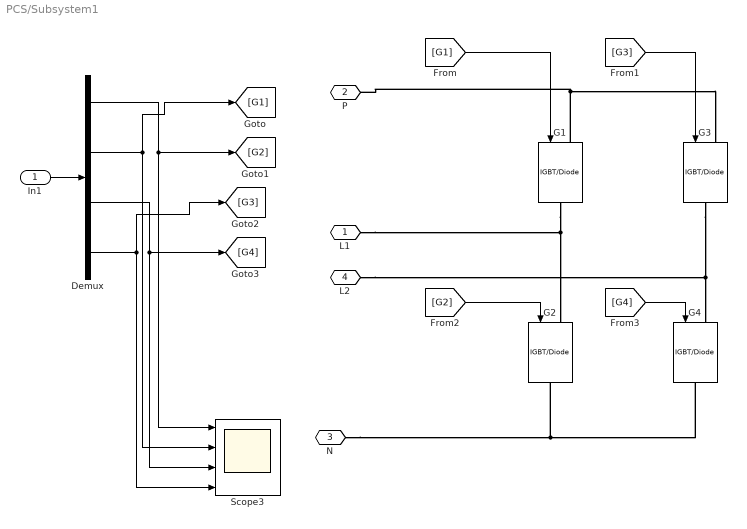
== system PCS/Subsystem1 ==
  In1 : Inport
  Demux : Demux
  G{1..4} (4 alike) : powerlib/Power Electronics/IGBT//Diode  Ron=1e-3  Rs=1e5  Cs=inf  Measurements=off
  Scope3 : Scope  NumInputPorts=4
  L1 : PMIOPort  Port=1  Side=Right
  P : PMIOPort  Port=2  Side=Left
  N : PMIOPort  Port=3  Side=Left
  L2 : PMIOPort  Port=4  Side=Right
  wires:
  In1/1 -> Demux/1
  [G1] -> G1/1
  Demux/1 -> [G2], Scope3/1
  Demux/2 -> [G1], Scope3/2
  Demux/4 -> [G3], Scope3/4
  [G3] -> G3/1
  [G2] -> G2/1
  [G4] -> G4/1
  Demux/3 -> [G4], Scope3/3
  connections:
  G1/RConn1 -- G2/LConn1 -- L1/RConn1
  G3/RConn1 -- L2/RConn1 -- G4/LConn1
  G1/LConn1 -- G3/LConn1 -- P/RConn1
  N/RConn1 -- G4/RConn1 -- G2/RConn1

== system PCS/Inv_Control/Alpha_Beta 1 ==
  abc : Inport
  Alpha : Fcn  Expr=(u[1]-0.5*u[2]-0.5*u[3])*2/3  SampleTime=Ts_PLL
  Beta : Fcn  Expr=(u[2]-u[3])*sqrt(3)/3  SampleTime=Ts_PLL
  Mux : Mux  Inputs=2
  Scope : Scope  NumInputPorts=2
  Alpha_Beta : Outport
  wires:
  abc/1 -> Beta/1, Alpha/1
  Mux/1 -> Alpha_Beta/1
  Alpha/1 -> Mux/1
  Beta/1 -> Mux/2

== system PCS/Inv_Control/Clack  ==
  abc : Inport
  Alpha : Fcn  Expr=(u[1]-0.5*u[2]-0.5*u[3])*2/3  SampleTime=Ts_PLL
  Beta : Fcn  Expr=(u[2]-u[3])*sqrt(3)/3  SampleTime=Ts_PLL
  Mux : Mux  Inputs=2
  Scope : Scope  NumInputPorts=2
  Alpha_Beta : Outport
  wires:
  abc/1 -> Beta/1, Alpha/1
  Mux/1 -> Alpha_Beta/1
  Alpha/1 -> Mux/1
  Beta/1 -> Mux/2

== system PCS/Inv_Control/DQ1 ==
  Alpha_Belta : Inport
  Sin_Cos : Inport  Port=2
  Mux : Mux  Inputs=2
  Mux1 : Mux  Inputs=2
  d : Fcn  Expr=(u[1]*u[4]+u[2]*u[3])  SampleTime=Ts_PLL
  q : Fcn  Expr=-u[1]*u[3]+u[2]*u[4]  SampleTime=Ts_PLL
  dq : Outport
  wires:
  q/1 -> Mux/2
  d/1 -> Mux/1
  Mux/1 -> dq/1
  Alpha_Belta/1 -> Mux1/1
  Sin_Cos/1 -> Mux1/2
  Mux1/1 -> d/1, q/1

== system PCS/Inv_Control/InvClack  ==
  Alpha_Beta : Inport
  Alpha : Fcn  Expr=u[1]  SampleTime=Ts_PLL
  Beta : Fcn  Expr=(sqrt(3)*u[2]-u[1])/2  SampleTime=Ts_PLL
  Beta1 : Fcn  Expr=(-sqrt(3)*u[2]-u[1])/2  SampleTime=Ts_PLL
  Mux : Mux  Inputs=3
  ABC : Outport
  wires:
  Alpha_Beta/1 -> Beta1/1, Beta/1, Alpha/1
  Mux/1 -> ABC/1
  Alpha/1 -> Mux/1
  Beta/1 -> Mux/2
  Beta1/1 -> Mux/3

== system PCS/Inv_Control/InvClack 1 ==
  Alpha_Beta : Inport
  Alpha : Fcn  Expr=u[1]  SampleTime=Ts_PLL
  Beta : Fcn  Expr=(sqrt(3)*u[2]-u[1])/2  SampleTime=Ts_PLL
  Beta1 : Fcn  Expr=(-sqrt(3)*u[2]-u[1])/2  SampleTime=Ts_PLL
  Mux : Mux  Inputs=3
  ABC : Outport
  wires:
  Alpha_Beta/1 -> Beta1/1, Beta/1, Alpha/1
  Mux/1 -> ABC/1
  Alpha/1 -> Mux/1
  Beta/1 -> Mux/2
  Beta1/1 -> Mux/3

== system PCS/Inv_Control/InvPark ==
  DQ : Inport
  Sin_Cos : Inport  Port=2
  Mux : Mux  Inputs=2
  Mux1 : Mux  Inputs=2
  Scope : Scope  NumInputPorts=2
  d : Fcn  Expr=(u[1]*u[4]-u[2]*u[3])  SampleTime=Ts_PLL
  q : Fcn  Expr=u[1]*u[3]+u[2]*u[4]  SampleTime=Ts_PLL
  Alpha_Belta : Outport
  wires:
  q/1 -> Mux/2
  d/1 -> Mux/1
  Mux/1 -> Alpha_Belta/1
  DQ/1 -> Mux1/1
  Sin_Cos/1 -> Mux1/2
  Mux1/1 -> d/1, q/1

== system PCS/Inv_Control/InvPark1 ==
  DQ : Inport
  Sin_Cos : Inport  Port=2
  Mux : Mux  Inputs=2
  Mux1 : Mux  Inputs=2
  Scope : Scope  NumInputPorts=2
  d : Fcn  Expr=(u[1]*u[4]-u[2]*u[3])  SampleTime=Ts_PLL
  q : Fcn  Expr=u[1]*u[3]+u[2]*u[4]  SampleTime=Ts_PLL
  Alpha_Belta : Outport
  wires:
  q/1 -> Mux/2
  d/1 -> Mux/1
  Mux/1 -> Alpha_Belta/1
  DQ/1 -> Mux1/1
  Sin_Cos/1 -> Mux1/2
  Mux1/1 -> d/1, q/1

== system PCS/Inv_Control/PI ==
  In : Inport
  Integrator : DiscreteIntegrator  gainval=1  SampleTime=Ts  ICPrevOutput=DiscIntNeverNeededParam  ICPrevScaledInput=DiscIntNeverNeededParam
  Kaw : Gain  DisableCoverage=on  Gain=Kaw  SampleTime=Ts
  Ki : Gain  DisableCoverage=on  Gain=Ki  SampleTime=Ts
  Kp : Gain  Gain=Kp  SampleTime=Ts
  Saturation : Saturate  UpperLimit=9*2*pi  LowerLimit=-9*2*pi  SampleTime=Ts
  Scope : Scope  NumInputPorts=2
  Scope1 : Scope  NumInputPorts=2
  Sum : Sum  Inputs=++|  SampleTime=Ts
  Sum1 : Sum  Inputs=|++  SampleTime=Ts
  Sum2 : Sum  Inputs=+-|  SampleTime=Ts
  out : Outport
  wires:
  In/1 -> Ki/1, Kp/1
  Integrator/1 -> Sum/2
  Kp/1 -> Sum/1
  Sum/1 -> Scope1/1, Sum2/2, Saturation/1, Scope/2
  Sum2/1 -> Kaw/1
  Saturation/1 -> Sum2/1, Scope/1, out/1
  Ki/1 -> Sum1/1
  Sum1/1 -> Integrator/1

== system PCS/Inv_Control/PI1 ==
  In : Inport
  Integrator : DiscreteIntegrator  gainval=1  SampleTime=Ts  ICPrevOutput=DiscIntNeverNeededParam  ICPrevScaledInput=DiscIntNeverNeededParam
  Kaw : Gain  DisableCoverage=on  Gain=Kaw  SampleTime=Ts
  Ki : Gain  DisableCoverage=on  Gain=Ki  SampleTime=Ts
  Kp : Gain  Gain=Kp  SampleTime=Ts
  Saturation : Saturate  UpperLimit=UpperLimit  LowerLimit=LowerLimit  SampleTime=Ts
  Scope : Scope  NumInputPorts=3
  Sum : Sum  Inputs=++|  SampleTime=Ts
  Sum1 : Sum  Inputs=|++  SampleTime=Ts
  Sum2 : Sum  Inputs=+-|  SampleTime=Ts
  out : Outport
  wires:
  In/1 -> Ki/1, Kp/1
  Integrator/1 -> Scope/3, Sum/2
  Kp/1 -> Scope/1, Sum/1
  Sum/1 -> Sum2/2, Saturation/1, Scope/2
  Sum2/1 -> Kaw/1
  Saturation/1 -> Sum2/1, out/1
  Ki/1 -> Sum1/1
  Sum1/1 -> Integrator/1
  Kaw/1 -> Sum1/2

== system PCS/Inv_Control/PI2 ==
  In : Inport
  In1 : Inport  Port=2
  In2 : Inport  Port=3
  Integrator : DiscreteIntegrator  gainval=1  SampleTime=Ts  ICPrevOutput=DiscIntNeverNeededParam  ICPrevScaledInput=DiscIntNeverNeededParam
  Kaw : Gain  DisableCoverage=on  Gain=Kaw  SampleTime=Ts
  Kaw1 : Gain  DisableCoverage=on  Gain=0.2861328125  SampleTime=125e-6
  Kaw5 : Gain  DisableCoverage=on  Gain=sqrt(3)/800  SampleTime=125e-6
  Ki : Gain  DisableCoverage=on  Gain=Ki  SampleTime=Ts
  Kp : Gain  Gain=Kp  SampleTime=Ts
  Saturation : Saturate  UpperLimit=UpperLimit  LowerLimit=LowerLimit  SampleTime=Ts
  Scope : Scope  NumInputPorts=2
  Sum : Sum  Inputs=++|  SampleTime=Ts
  Sum1 : Sum  Inputs=|++  SampleTime=Ts
  Sum2 : Sum  Inputs=+-|  SampleTime=Ts
  Sum3 : Sum  Inputs=-+|  SampleTime=Ts
  Sum4 : Sum  Inputs=-+|  SampleTime=Ts
  out : Outport
  wires:
  In/1 -> Ki/1, Kp/1
  Integrator/1 -> Sum/2
  Kp/1 -> Sum/1
  Sum2/1 -> Kaw/1
  Saturation/1 -> Sum2/1, Scope/1, out/1
  Ki/1 -> Sum1/1
  Sum1/1 -> Integrator/1
  In1/1 -> Kaw1/1
  Sum/1 -> Sum3/2
  Sum3/1 -> Kaw5/1
  Kaw1/1 -> Sum3/1
  Kaw5/1 -> Sum4/2
  In2/1 -> Sum4/1
  Sum4/1 -> Sum2/2, Saturation/1
  Kaw/1 -> Sum1/2

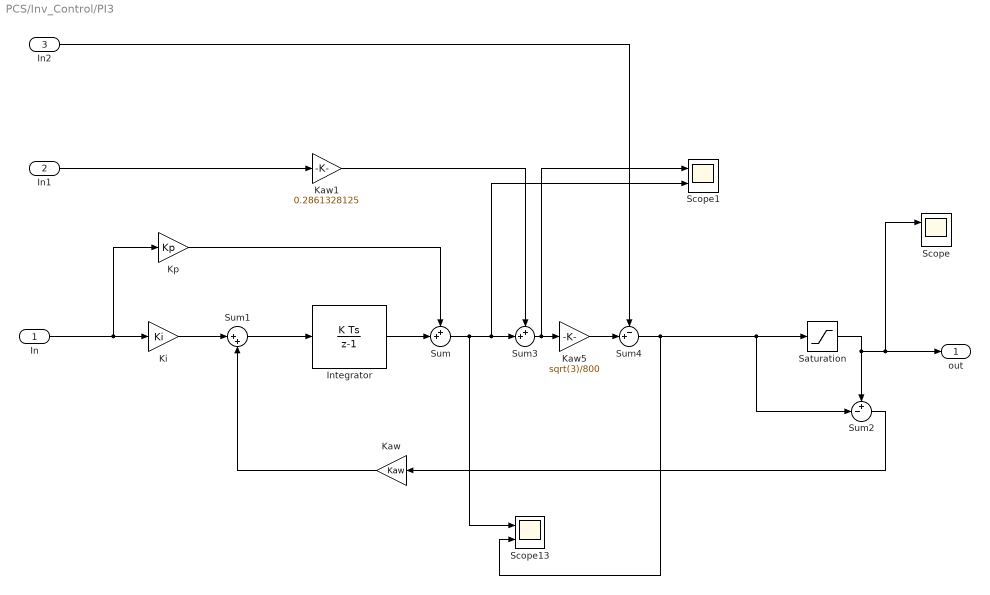
== system PCS/Inv_Control/PI3 ==
  In : Inport
  In1 : Inport  Port=2
  In2 : Inport  Port=3
  Integrator : DiscreteIntegrator  gainval=1  SampleTime=Ts  ICPrevOutput=DiscIntNeverNeededParam  ICPrevScaledInput=DiscIntNeverNeededParam
  Kaw : Gain  DisableCoverage=on  Gain=Kaw  SampleTime=Ts
  Kaw1 : Gain  DisableCoverage=on  Gain=0.2861328125  SampleTime=125e-6
  Kaw5 : Gain  DisableCoverage=on  Gain=sqrt(3)/800  SampleTime=125e-6
  Ki : Gain  DisableCoverage=on  Gain=Ki  SampleTime=Ts
  Kp : Gain  Gain=Kp  SampleTime=Ts
  Saturation : Saturate  UpperLimit=UpperLimit  LowerLimit=LowerLimit  SampleTime=Ts
  Scope : Scope  NumInputPorts=2
  Scope1 : Scope  NumInputPorts=2
  Scope13 : Scope  NumInputPorts=2
  Sum : Sum  Inputs=++|  SampleTime=Ts
  Sum1 : Sum  Inputs=|++  SampleTime=Ts
  Sum2 : Sum  Inputs=+-|  SampleTime=Ts
  Sum3 : Sum  Inputs=++|  SampleTime=Ts
  Sum4 : Sum  Inputs=-+|  SampleTime=Ts
  out : Outport
  wires:
  In/1 -> Ki/1, Kp/1
  Integrator/1 -> Sum/2
  Kp/1 -> Sum/1
  Sum2/1 -> Kaw/1
  Saturation/1 -> Sum2/1, Scope/1, out/1
  Ki/1 -> Sum1/1
  Sum1/1 -> Integrator/1
  In1/1 -> Kaw1/1
  Sum/1 -> Scope13/1, Scope1/2, Sum3/2
  Sum3/1 -> Scope1/1, Kaw5/1
  Kaw1/1 -> Sum3/1
  Kaw5/1 -> Sum4/2
  In2/1 -> Sum4/1
  Sum4/1 -> Scope13/2, Sum2/2, Saturation/1
  Kaw/1 -> Sum1/2

== system PCS/Inv_Control/Park ==
  Alpha_Belta : Inport
  Sin_Cos : Inport  Port=2
  Mux : Mux  Inputs=2
  Mux1 : Mux  Inputs=2
  Scope : Scope  NumInputPorts=2
  d : Fcn  Expr=(u[1]*u[4]+u[2]*u[3])  SampleTime=Ts_PLL
  q : Fcn  Expr=-u[1]*u[3]+u[2]*u[4]  SampleTime=Ts_PLL
  dq : Outport
  wires:
  q/1 -> Mux/2
  d/1 -> Mux/1
  Mux/1 -> dq/1
  Alpha_Belta/1 -> Mux1/1
  Sin_Cos/1 -> Mux1/2
  Mux1/1 -> d/1, q/1

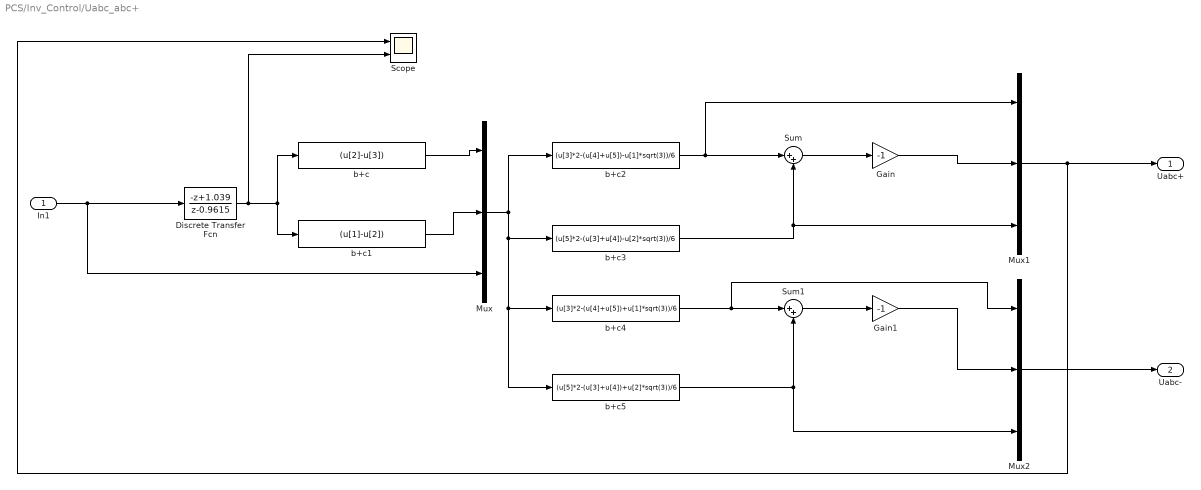
== system PCS/Inv_Control/Uabc_abc+ ==
  In1 : Inport
  Discrete Transfer Fcn : DiscreteTransferFcn  Numerator=[-1 1.039]  Denominator=[1 -0.9615]  SampleTime=Ts_PLL
  Gain : Gain  Gain=-1  SampleTime=Ts_PLL
  Gain1 : Gain  Gain=-1  SampleTime=Ts_PLL
  Mux : Mux  Inputs=3
  Mux1 : Mux  Inputs=3
  Mux2 : Mux  Inputs=3
  Scope : Scope  NumInputPorts=2
  Sum : Sum  Inputs=|++
  Sum1 : Sum  Inputs=|++
  b+c : Fcn  Expr=(u[2]-u[3])  SampleTime=Ts_PLL
  b+c1 : Fcn  Expr=(u[1]-u[2])  SampleTime=Ts_PLL
  b+c2 : Fcn  Expr=(u[3]*2-(u[4]+u[5])-u[1]*sqrt(3))/6  SampleTime=Ts_PLL
  b+c3 : Fcn  Expr=(u[5]*2-(u[3]+u[4])-u[2]*sqrt(3))/6  SampleTime=Ts_PLL
  b+c4 : Fcn  Expr=(u[3]*2-(u[4]+u[5])+u[1]*sqrt(3))/6  SampleTime=Ts_PLL
  b+c5 : Fcn  Expr=(u[5]*2-(u[3]+u[4])+u[2]*sqrt(3))/6  SampleTime=Ts_PLL
  Uabc+ : Outport
  Uabc- : Outport  Port=2
  wires:
  In1/1 -> Discrete Transfer Fcn/1, Mux/3
  Discrete Transfer Fcn/1 -> Scope/2, b+c1/1, b+c/1
  b+c/1 -> Mux/1
  b+c1/1 -> Mux/2
  Mux/1 -> b+c5/1, b+c4/1, b+c3/1, b+c2/1
  b+c2/1 -> Mux1/1, Sum/1
  Sum/1 -> Gain/1
  b+c4/1 -> Mux2/1, Sum1/1
  b+c5/1 -> Sum1/2, Mux2/3
  Sum1/1 -> Gain1/1
  Gain/1 -> Mux1/2
  Mux2/1 -> Uabc-/1
  Mux1/1 -> Scope/1, Uabc+/1
  b+c3/1 -> Mux1/3, Sum/2
  Gain1/1 -> Mux2/2

== system PCS/Inv_Control/Udc_PN ==
  In1 : Inport
  Alpha : Fcn  Expr=u[1]+u[2]  SampleTime=Ts_PLL
  Alpha1 : Fcn  Expr=u[1]-u[2]  SampleTime=Ts_PLL
  Udc_Fdb : Outport
  Udc_diff : Outport  Port=2
  wires:
  In1/1 -> Alpha1/1, Alpha/1
  Alpha/1 -> Udc_Fdb/1
  Alpha1/1 -> Udc_diff/1

== system PCS/Modu1/PI ==
  In : Inport
  Integrator : DiscreteIntegrator  gainval=1  SampleTime=Ts  ICPrevOutput=DiscIntNeverNeededParam  ICPrevScaledInput=DiscIntNeverNeededParam
  Kaw : Gain  DisableCoverage=on  Gain=Kaw  SampleTime=Ts
  Ki : Gain  DisableCoverage=on  Gain=Ki  SampleTime=Ts
  Kp : Gain  Gain=Kp  SampleTime=Ts
  Saturation : Saturate  UpperLimit=UpperLimit  LowerLimit=LowerLimit  SampleTime=Ts
  Scope : Scope  NumInputPorts=2
  Sum : Sum  Inputs=++|  SampleTime=Ts
  Sum1 : Sum  Inputs=|++  SampleTime=Ts
  Sum2 : Sum  Inputs=+-|  SampleTime=Ts
  out : Outport
  wires:
  In/1 -> Ki/1, Kp/1
  Integrator/1 -> Scope/2, Sum/2
  Kp/1 -> Sum/1
  Sum/1 -> Sum2/2, Saturation/1
  Sum2/1 -> Kaw/1
  Saturation/1 -> Sum2/1, Scope/1, out/1
  Ki/1 -> Sum1/1
  Sum1/1 -> Integrator/1
  Kaw/1 -> Sum1/2

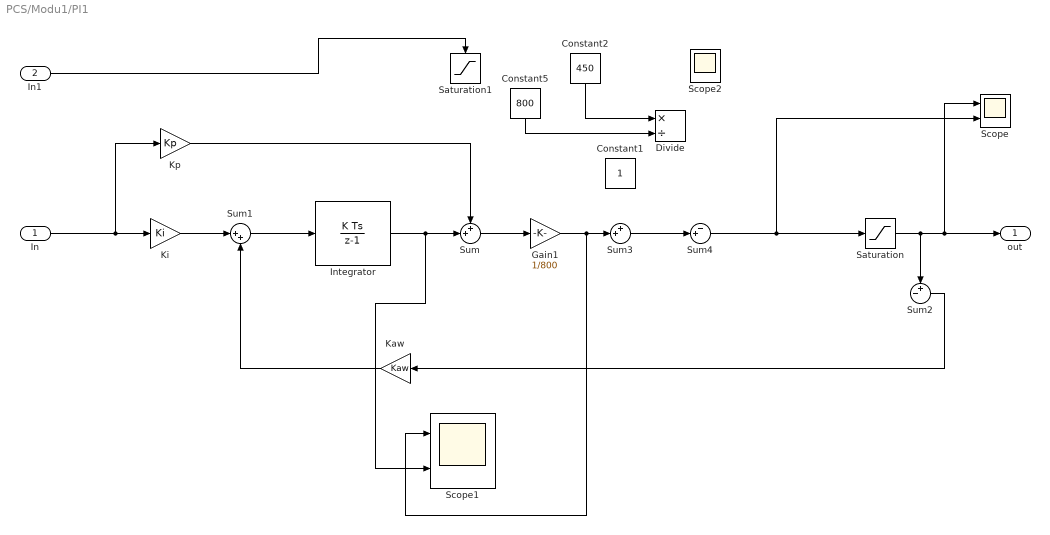
== system PCS/Modu1/PI1 ==
  In : Inport
  In1 : Inport  Port=2
  Constant1 : Constant
  Constant2 : Constant  Value=450
  Constant5 : Constant  Value=800
  Divide : Product  Inputs=*/
  Gain1 : Gain  Gain=1/800  SampleTime=Ts_Dc
  Integrator : DiscreteIntegrator  gainval=1  SampleTime=Ts  ICPrevOutput=DiscIntNeverNeededParam  ICPrevScaledInput=DiscIntNeverNeededParam
  Kaw : Gain  DisableCoverage=on  Gain=Kaw  SampleTime=Ts
  Ki : Gain  DisableCoverage=on  Gain=Ki  SampleTime=Ts
  Kp : Gain  Gain=Kp  SampleTime=Ts
  Saturation : Saturate  UpperLimit=UpperLimit  LowerLimit=LowerLimit  SampleTime=Ts
  Saturation1 : Saturate  UpperLimit=950  LowerLimit=100  SampleTime=Ts
  Scope : Scope  NumInputPorts=2
  Scope1 : Scope  NumInputPorts=2
  Scope2 : Scope  NumInputPorts=2
  Sum : Sum  Inputs=++|  SampleTime=Ts
  Sum1 : Sum  Inputs=|++  SampleTime=Ts
  Sum2 : Sum  Inputs=+-|  SampleTime=Ts
  Sum3 : Sum  Inputs=++|  SampleTime=Ts
  Sum4 : Sum  Inputs=-+|  SampleTime=Ts
  out : Outport
  wires:
  Sum1/1 -> Integrator/1
  Ki/1 -> Sum1/1
  Saturation/1 -> out/1, Scope/1, Sum2/1
  Sum2/1 -> Kaw/1
  Kp/1 -> Sum/1
  Integrator/1 -> Scope1/2, Sum/2
  In/1 -> Kp/1, Ki/1
  In1/1 -> Saturation1/1
  Sum/1 -> Gain1/1
  Gain1/1 -> Scope1/1, Sum3/2
  Sum3/1 -> Sum4/2
  Sum4/1 -> Scope/2, Saturation/1
  Constant5/1 -> Divide/2
  Constant2/1 -> Divide/1
  Kaw/1 -> Sum1/2

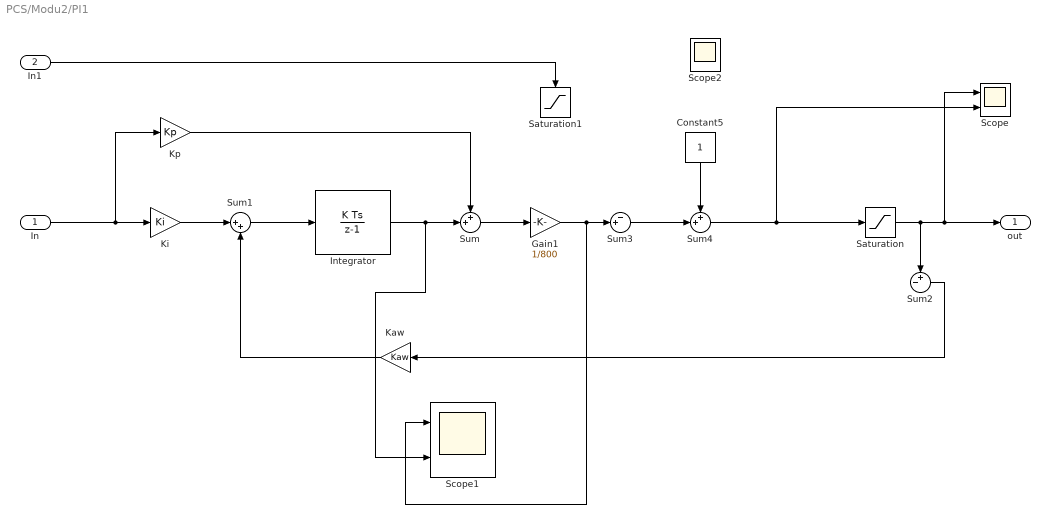
== system PCS/Modu2/PI1 ==
  In : Inport
  In1 : Inport  Port=2
  Constant5 : Constant
  Gain1 : Gain  Gain=1/800  SampleTime=Ts_Dc
  Integrator : DiscreteIntegrator  gainval=1  SampleTime=Ts  ICPrevOutput=DiscIntNeverNeededParam  ICPrevScaledInput=DiscIntNeverNeededParam
  Kaw : Gain  DisableCoverage=on  Gain=Kaw  SampleTime=Ts
  Ki : Gain  DisableCoverage=on  Gain=Ki  SampleTime=Ts
  Kp : Gain  Gain=Kp  SampleTime=Ts
  Saturation : Saturate  UpperLimit=UpperLimit  LowerLimit=LowerLimit  SampleTime=Ts
  Saturation1 : Saturate  UpperLimit=1000  LowerLimit=0  SampleTime=Ts
  Scope : Scope  NumInputPorts=2
  Scope1 : Scope  NumInputPorts=2
  Scope2 : Scope  NumInputPorts=2
  Sum : Sum  Inputs=++|  SampleTime=Ts
  Sum1 : Sum  Inputs=|++  SampleTime=Ts
  Sum2 : Sum  Inputs=+-|  SampleTime=Ts
  Sum3 : Sum  Inputs=-+|  SampleTime=Ts
  Sum4 : Sum  Inputs=++|  SampleTime=Ts
  out : Outport
  wires:
  Sum1/1 -> Integrator/1
  Ki/1 -> Sum1/1
  Saturation/1 -> out/1, Scope/1, Sum2/1
  Sum2/1 -> Kaw/1
  Kp/1 -> Sum/1
  Integrator/1 -> Scope1/2, Sum/2
  In/1 -> Kp/1, Ki/1
  In1/1 -> Saturation1/1
  Sum/1 -> Gain1/1
  Gain1/1 -> Scope1/1, Sum3/2
  Sum3/1 -> Sum4/2
  Sum4/1 -> Scope/2, Saturation/1
  Constant5/1 -> Sum4/1
  Kaw/1 -> Sum1/2

== system PCS/NPC/Sa ==
  Sa1 : powerlib/Power Electronics/IGBT//Diode  Ron=1e-3  Rs=1e5  Cs=inf  Measurements=off
  Sa2 : powerlib/Power Electronics/IGBT//Diode  Ron=1e-3  Rs=1e6  Cs=inf  Measurements=on
  Sa3 : powerlib/Power Electronics/IGBT//Diode  Ron=1e-3  Rs=1e6  Cs=inf  Measurements=on
  Sa4 : powerlib/Power Electronics/IGBT//Diode  Ron=1e-3  Rs=1e6  Cs=inf  Measurements=on
  P : PMIOPort  Port=1  Side=Right
  Ua : PMIOPort  Port=2  Side=Left
  O : PMIOPort  Port=3  Side=Right
  N : PMIOPort  Port=4  Side=Right
  wires:
  [Sa1_A] -> Sa1/1
  [Sa2_A] -> Sa2/1
  [Sa3_A] -> Sa3/1
  [Sa4_A] -> Sa4/1
  connections:
  Sa1/RConn1 -- Ua/RConn1 -- Sa4/LConn1 -- Sa3/LConn1
  N/RConn1 -- Sa4/RConn1
  O/RConn1 -- Sa2/LConn1
  P/RConn1 -- Sa1/LConn1
  Sa2/RConn1 -- Sa3/RConn1

== system PCS/NPC/Sb ==
  Sb{1..4} (4 alike) : powerlib/Power Electronics/IGBT//Diode  Ron=1e-3  Rs=1e6  Cs=inf  Measurements=on
  P : PMIOPort  Port=1  Side=Right
  Ub : PMIOPort  Port=2  Side=Left
  O : PMIOPort  Port=3  Side=Right
  N : PMIOPort  Port=4  Side=Right
  wires:
  [Sb4_B] -> Sb4/1
  [Sb3_B] -> Sb3/1
  [Sb2_B] -> Sb2/1
  [Sb1_B] -> Sb1/1
  connections:
  Sb2/RConn1 -- Sb3/RConn1
  P/RConn1 -- Sb1/LConn1
  O/RConn1 -- Sb2/LConn1
  N/RConn1 -- Sb4/RConn1
  Sb4/LConn1 -- Sb3/LConn1 -- Sb1/RConn1 -- Ub/RConn1

== system PCS/NPC/Sc ==
  Sc1 : powerlib/Power Electronics/IGBT//Diode  Ron=1e-3  Rs=1e6  Cs=inf  Measurements=off
  Sc2 : powerlib/Power Electronics/IGBT//Diode  Ron=1e-3  Rs=1e6  Cs=inf  Measurements=on
  Sc3 : powerlib/Power Electronics/IGBT//Diode  Ron=1e-3  Rs=1e6  Cs=inf  Measurements=on
  Sc4 : powerlib/Power Electronics/IGBT//Diode  Ron=1e-3  Rs=1e6  Cs=inf  Measurements=off
  P : PMIOPort  Port=1  Side=Right
  Uc : PMIOPort  Port=2  Side=Left
  O : PMIOPort  Port=3  Side=Right
  N : PMIOPort  Port=4  Side=Right
  wires:
  [Sc1_C] -> Sc1/1
  [Sc2_C] -> Sc2/1
  [Sc3_C] -> Sc3/1
  [Sc4_C] -> Sc4/1
  connections:
  Sc1/RConn1 -- Uc/RConn1 -- Sc4/LConn1 -- Sc3/LConn1
  N/RConn1 -- Sc4/RConn1
  O/RConn1 -- Sc2/LConn1
  P/RConn1 -- Sc1/LConn1
  Sc2/RConn1 -- Sc3/RConn1
